simulink model "WSW"  (R2022b)
settings: Solver=FixedStepAuto  StartTime=0.0  StopTime=10.0  RelTol=1e-3
settings Model: Creator=MAAM  LastModifiedBy=MAAM
settings OptimizationCC: DefaultParameterBehavior=Inlined  UseDivisionForNetSlopeComputation=on  GainParamInheritBuiltInType=on  UseFloatMulNetSlope=on  InlineInvariantSignals=on  PassReuseOutputArgsAs=Individual arguments  ZeroExternalMemoryAtStartup=off  ZeroInternalMemoryAtStartup=off  NoFixptDivByZeroProtection=on  EfficientFloat2IntCast=on  LifeSpan=1  OptimizeBlockOrder=speed  DifferentSizesBufferReuse=on  EfficientTunableParamExpr=on
settings DebuggingCC: ParameterTunabilityLossMsg=error
settings HardwareCC: ProdLongLongMode=on
settings SFSimCC: MATLABDynamicMemAlloc=off
settings RTWCC: Description=Embedded Coder  SystemTargetFile=ert.tlc  TemplateMakefile=ert_default_tmf  CreateSILPILBlock=SIL
settings CodeAppCC: ForceParamTrailComments=on  IgnoreCustomStorageClasses=off  OperatorAnnotations=on  SimulinkDataObjDesc=on  SFDataObjDesc=on  CustomSymbolStrGlobalVar=rt$N$M  CustomSymbolStrType=$N$M  CustomSymbolStrFcn=$N$M$F  CustomSymbolStrMacro=$N$M  InsertBlockDesc=on
settings ERTTargetCC: TargetLangStandard=C99 (ISO)  GenerateSampleERTMain=on  IncludeMdlTerminateFcn=off  CombineSignalStateStructs=on  SuppressErrorStatus=on  SupportAbsoluteTime=off  PurelyIntegerCode=on  SupportNonFinite=off  SupportComplex=off  InlinedParameterPlacement=NonHierarchical  ERTCustomFileTemplate=example_file_process.tlc  ERTFilePackagingFormat=CompactWithDataFile

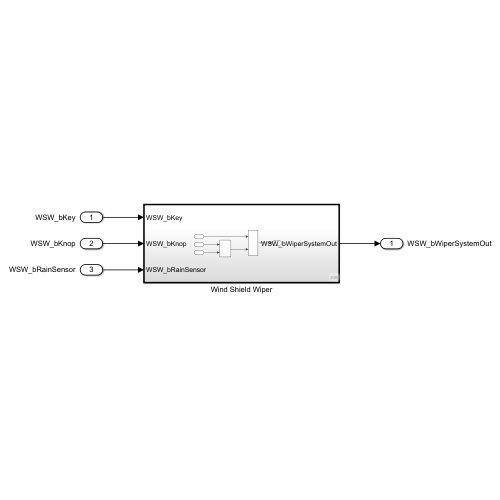
[thumbnail: Simulink's stored preview of the top-level diagram]
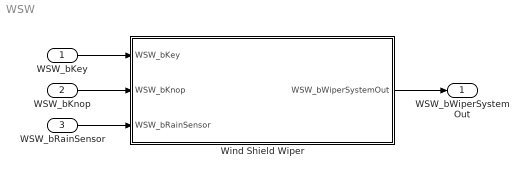
== system WSW ==
  WSW_bKey : Inport  OutDataTypeStr=boolean
  WSW_bKnop : Inport  Port=2  OutDataTypeStr=boolean
  WSW_bRainSensor : Inport  Port=3  OutDataTypeStr=boolean
  Wind Shield Wiper : Subsystem  TreatAsAtomicUnit=on
  WSW_bWiperSystemOut : Outport  OutDataTypeStr=boolean
  wires:
  WSW_bKey/1 -> Wind Shield Wiper/1(WSW_bKey)
  WSW_bKnop/1 -> Wind Shield Wiper/2(WSW_bKnop)
  WSW_bRainSensor/1 -> Wind Shield Wiper/3(WSW_bRainSensor)
  Wind Shield Wiper/1(WSW_bWiperSystemOut) -> WSW_bWiperSystemOut/1

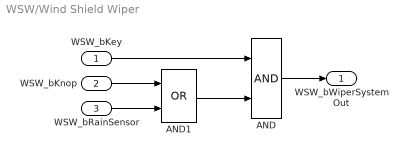
== system WSW/Wind Shield Wiper ==
  WSW_bKey : Inport  OutDataTypeStr=boolean
  WSW_bKnop : Inport  Port=2  OutDataTypeStr=boolean
  WSW_bRainSensor : Inport  Port=3  OutDataTypeStr=boolean
  AND : Logic  AllPortsSameDT=off  OutDataTypeStr=boolean
  AND1 : Logic  Operator=OR  AllPortsSameDT=off  OutDataTypeStr=boolean
  WSW_bWiperSystemOut : Outport  OutDataTypeStr=boolean
  wires:
  WSW_bKnop/1 -> AND1/1
  AND1/1 -> AND/2
  WSW_bRainSensor/1 -> AND1/2
  WSW_bKey/1 -> AND/1
  AND/1 -> WSW_bWiperSystemOut/1
